simulink model "FltDiagLmt"  (R2024b)
settings: configuration reference "BMS_Sw_CodeGenConfig" (kept outside this file)
undefined symbols (not defined in the file): Battery, OverCellVoltageLimit, OverCurDisLmt, ts
settings Model: DataDictionary=DD_CurrPowerLimCalc.sldd  EnableAccessToBaseWorkspace=off  ExtModeTrigDuration=5  Creator=cpatel  LastModifiedBy=18811
settings ConfigSetRef: SourceName=BMS_Sw_CodeGenConfig

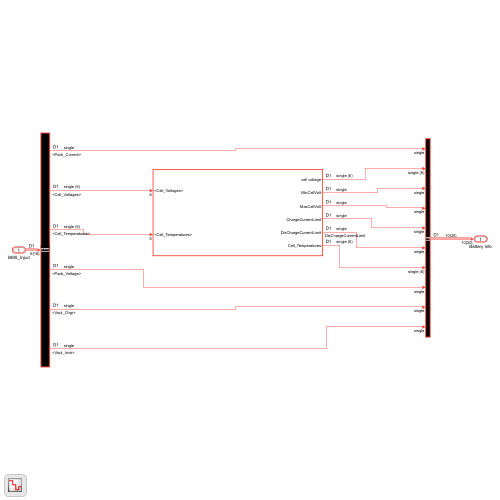
[thumbnail: Simulink's stored preview of the top-level diagram]
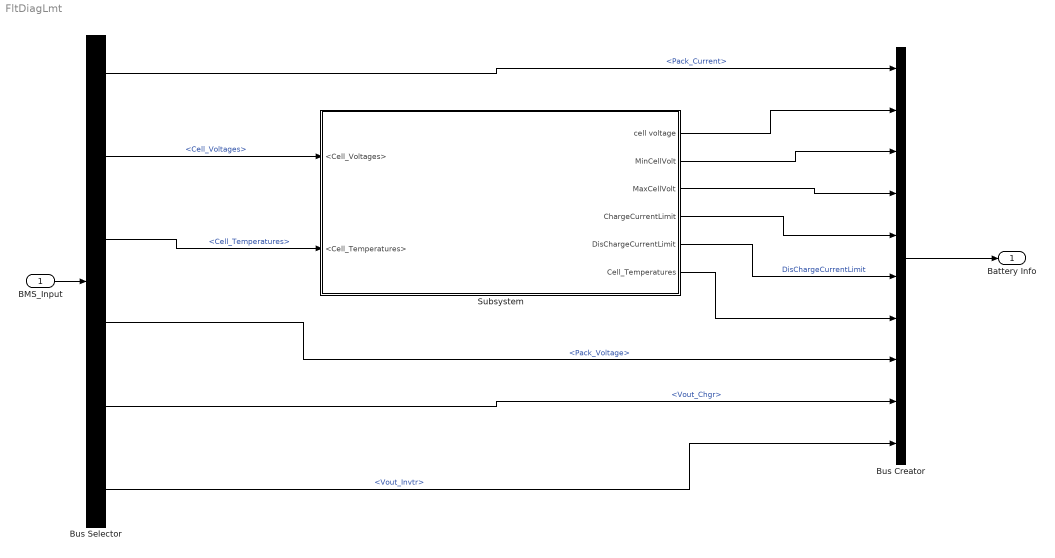
== system FltDiagLmt ==
  BMS_Input : Inport  OutDataTypeStr=Bus: BMS_Input
  Bus Creator : BusCreator  Inputs=10  OutDataTypeStr=Bus: Battery_Info
      settings: InheritFromInputs=off
  Bus Selector : BusSelector  OutputSignals=Pack_Current,Cell_Voltages,Cell_Temperatures,Pack_Voltage,Vout_Chgr,Vout_Invtr
  Subsystem : Subsystem
  Battery Info : Outport  OutDataTypeStr=Bus: Battery_Info
  wires:
  BMS_Input/1 -> Bus Selector/1
  Bus Creator/1 -> Battery Info/1
  Bus Selector/1 -> Bus Creator/1  "<Pack_Current>"
  Bus Selector/2 -> Subsystem/1(<Cell_Voltages>)  "<Cell_Voltages>"
  Bus Selector/3 -> Subsystem/2(<Cell_Temperatures>)  "<Cell_Temperatures>"
  Subsystem/2(MinCellVolt) -> Bus Creator/3
  Subsystem/3(MaxCellVolt) -> Bus Creator/4
  Subsystem/4(ChargeCurrentLimit) -> Bus Creator/5
  Bus Selector/4 -> Bus Creator/8  "<Pack_Voltage>"
  Bus Selector/5 -> Bus Creator/9  "<Vout_Chgr>"
  Bus Selector/6 -> Bus Creator/10  "<Vout_Invtr>"
  Subsystem/5(DisChargeCurrentLimit) -> Bus Creator/6  "DisChargeCurrentLimit"
  Subsystem/1(cell voltage) -> Bus Creator/2
  Subsystem/6(Cell_Temperatures) -> Bus Creator/7

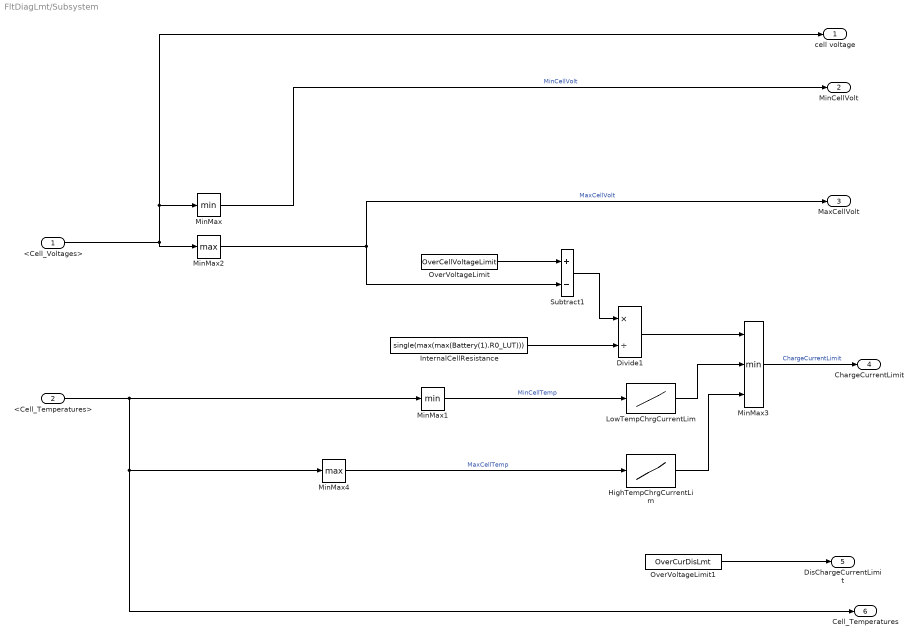
== system FltDiagLmt/Subsystem ==
  <Cell_Voltages> : Inport
  <Cell_Temperatures> : Inport  Port=2
  Divide1 : Product  Inputs=*/
  HighTempChrgCurrentLim : Lookup_n-D  NumberOfTableDimensions=1  BreakpointsForDimension1=273.15+[-30:1:70]  Table=50*(1-tanh(273.15+[-30:1:70]-273.15-50))/2  InternalRulePriority=Speed  RndMeth=Simplest
  InternalCellResistance : Constant  Value=single(max(max(Battery(1).R0_LUT)))  OutDataTypeStr=single  SampleTime=ts
  LowTempChrgCurrentLim : Lookup_n-D  NumberOfTableDimensions=1  BreakpointsForDimension1=273.15+[-30:1:70]  Table=50*(1+tanh(273.15+[-30:1:70]-(273.15)))/2  InternalRulePriority=Speed  RndMeth=Simplest
  MinMax : MinMax
  MinMax1 : MinMax
  MinMax2 : MinMax  Function=max
  MinMax3 : MinMax  Inputs=3
  MinMax4 : MinMax  Function=max
  OverVoltageLimit : Constant  Value=OverCellVoltageLimit  OutDataTypeStr=single  SampleTime=ts
  OverVoltageLimit1 : Constant  Value=OverCurDisLmt  OutDataTypeStr=single  SampleTime=ts
  Subtract1 : Sum  Inputs=+-
  cell voltage : Outport
  MinCellVolt : Outport  Port=2
  MaxCellVolt : Outport  Port=3
  ChargeCurrentLimit : Outport  Port=4
  DisChargeCurrentLimit : Outport  Port=5
  Cell_Temperatures : Outport  Port=6
  wires:
  InternalCellResistance/1 -> Divide1/2
  MinMax1/1 -> LowTempChrgCurrentLim/1  "MinCellTemp"
  HighTempChrgCurrentLim/1 -> MinMax3/3
  Subtract1/1 -> Divide1/1
  <Cell_Voltages>/1 -> cell voltage/1, MinMax/1, MinMax2/1
  LowTempChrgCurrentLim/1 -> MinMax3/2
  MinMax/1 -> MinCellVolt/1  "MinCellVolt"
  Divide1/1 -> MinMax3/1
  OverVoltageLimit/1 -> Subtract1/1
  MinMax2/1 -> MaxCellVolt/1, Subtract1/2  "MaxCellVolt"
  <Cell_Temperatures>/1 -> MinMax1/1, Cell_Temperatures/1, MinMax4/1
  MinMax4/1 -> HighTempChrgCurrentLim/1  "MaxCellTemp"
  MinMax3/1 -> ChargeCurrentLimit/1  "ChargeCurrentLimit"
  OverVoltageLimit1/1 -> DisChargeCurrentLimit/1
